simulink model "MPCSimulationSlowest"  (Simulink 9.1)
settings: Solver=ode45  StartTime=0.0  StopTime=10  RelTol=1e-3  EnableMultiTasking=on
values from neighbouring files (symbols this model uses):
  A = plant.A    [MPCController.m]    (also in SlowMPCController.m = Plant.A; Untitled.m = [0,0,0;0,0,0;-1,1,0]; setupsimulation.m = [0,0;1,0])
  B = plant.B    [MPCController.m]    (also in SlowMPCController.m = Plant.B; Untitled.m = [0;1;0]; setupsimulation.m = [1;0])
  C = plant.C    [MPCController.m]    (also in SlowMPCController.m = Plant.C; Untitled.m = [0,0,1]; setupsimulation.m = [0,1])
  Ts = 0.5    [MPCController.m]    (also in SlowMPCController.m = 0.1; Untitled.m; setupsimulation.m = 0.1)
  x0 = [20;22;-80]    [Untitled.m]    (also in setupsimulation.m = [1;1])
undefined symbols (not defined in the file or in its folder): SlowestMPCController
settings Model: Creator=johanl  LastModifiedBy=HP
settings DataIOCC: LimitDataPoints=on  SignalLoggingSaveFormat=ModelDataLogs
settings OptimizationCC: ExpressionDepthLimit=2147483647
settings DebuggingCC: SolverPrmCheckMsg=warning  FcnCallInpInsideContextMsg=warning  StateNameClashWarn=warning
settings GRTTargetCC: GeneratePreprocessorConditionals=Disable all  CombineOutputUpdateFcns=on  GRTInterface=off

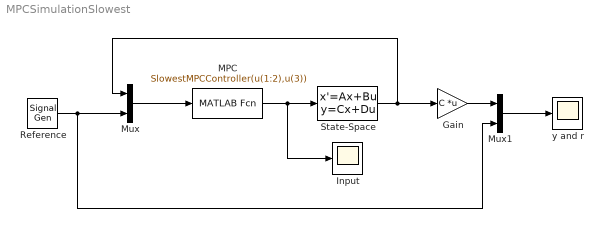
== system MPCSimulationSlowest ==
  Gain : Gain  Gain=C  Multiplication=Matrix(K*u)
  Input : Scope
  MPC : MATLABFcn  MATLABFcn=SlowestMPCController(u(1:2),u(3))  SampleTime=Ts
  Mux : Mux  Inputs=2
  Mux1 : Mux  Inputs=2
  Reference : SignalGenerator  WaveForm=square  Frequency=0.2
  State-Space : StateSpace  A=A  B=B  C=eye(2)  D=zeros(2,1)  InitialCondition=x0
  y and r : Scope
  wires:
  State-Space/1 -> Mux/1, Gain/1
  MPC/1 -> State-Space/1, Input/1
  Mux/1 -> MPC/1
  Reference/1 -> Mux/2, Mux1/2
  Gain/1 -> Mux1/1
  Mux1/1 -> y and r/1
